simulink model "F16NolinearModel"  (R2013a)
settings: Solver=ode45  StartTime=0.0  StopTime=10  RelTol=1e-3
values from neighbouring files (symbols this model uses):
  alpha0 = trim_state(8)*180/pi    [F16LinmodTestData.m]    (also in F16NolinearModelInitialData.m; F16NolinearModelRemoveWindControlData_low.m = 0; testdata.m)
  b_ref = 9.144    [F16LinmodTestData.m]    (also in F16NolinearModelInitialData.m; F16NolinearModelRemoveWindControlData_low.m = 30; testdata.m = 30)
  dLEF = 0    [F16Data.mat]    (also in F16LinmodTestData.m; F16NolinearModelInitialData.m; F16NolinearModelRemoveWindControlData_low.m; F16hi_7500_394_all.mat)
  fi_flag = 0    [F16LinmodTestData.m]    (also in F16NolinearModelInitialData.m = 1; F16NolinearModelRemoveWindControlData_low.m; testdata.m = 1)
  mass = 636.94*14.59428    (= 9295.6807032)    [F16LinmodTestData.m]    (also in F16NolinearModelInitialData.m; F16NolinearModelRemoveWindControlData_low.m = 636.94; testdata.m = 636.94)
  q = input('Enter the pull-up rate (deg/s):  ')    [trim_F16.m]
  r = input('Enter the turning rate (deg/s):  ')    [trim_F16.m]
  trim_ail = 0.00874607850103852    (= 0.00874607850104)    [F16LinmodTestData.m]    (also in F16NolinearModelInitialData.m; F16NolinearModelRemoveWindControlData_low.m = -1.24450697103e-10; testdata.m; trim_F16.m = UX(4))
  trim_control = [trim_thrust;trim_ele;trim_ail;trim_rud]    [F16LinmodTestData.m]    (also in F16NolinearModelInitialData.m = [trim_thrust,trim_ele,trim_ail,trim_rud]; F16NolinearModelRemoveWindControlData_low.m; runLINF16sim.m = trim_control_lo; testdata.m)
  trim_ele = -2.97973164860638    (= -2.97973164861)    [F16LinmodTestData.m]    (also in F16NolinearModelInitialData.m; F16NolinearModelRemoveWindControlData_low.m = -1.5494258131; testdata.m; trim_F16.m = UX(2))
  trim_rud = 0.0680302158182712    (= 0.0680302158183)    [F16LinmodTestData.m]    (also in F16NolinearModelInitialData.m; F16NolinearModelRemoveWindControlData_low.m = -4.77959844983e-09; testdata.m; trim_F16.m = UX(5))
  trim_thrust = 500    [F16LinmodTestData.m]    (also in F16NolinearModelInitialData.m = 2279.08519955; F16NolinearModelRemoveWindControlData_low.m = -206727.459732; runLINF16sim.m = trim_thrust_lo; testdata.m = 2279.08519955)
  x_cg = 0.09144    [F16LinmodTestData.m]    (also in F16NolinearModelInitialData.m; F16NolinearModelRemoveWindControlData_low.m = 3.962; testdata.m = 3.962)
  x_ref = 0.10668    [F16LinmodTestData.m]    (also in F16NolinearModelInitialData.m; F16NolinearModelRemoveWindControlData_low.m = 3.396; testdata.m = 3.396)
undefined symbols (not defined in the file or in its folder): F, Light, MIL
libraries: aerolibasang x3, aerolibwind2 x3, aerolib6dof2 x1, aerolibconvert2 x1, aerolibatmos2 x1, aerolibgravity2 x1, aerolibadyn x1
settings Model: Creator=Dai  LastModifiedBy=Dai

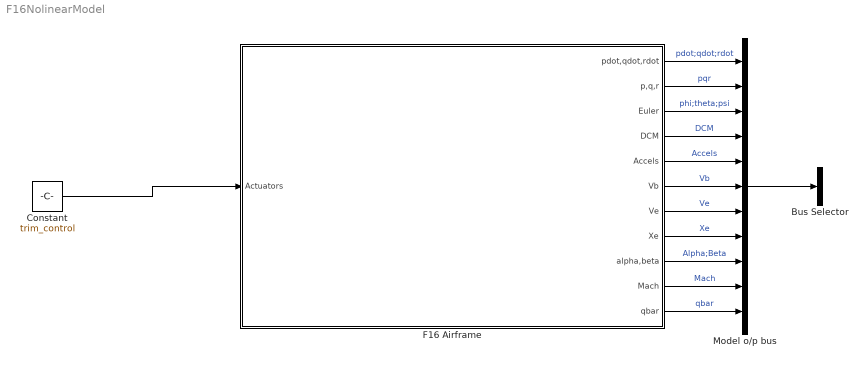
== system F16NolinearModel ==
  Bus Selector : BusSelector  OutputSignals=pdot;qdot;rdot,pqr
  Constant : Constant  Value=trim_control
  F16 Airframe : Subsystem
  Model o/p bus : BusCreator  Inputs=11
  wires:
  F16 Airframe/1(pdot,qdot,rdot) -> Model o/p bus/1  "pdot;qdot;rdot"
  F16 Airframe/2(p,q,r) -> Model o/p bus/2  "pqr"
  F16 Airframe/3(Euler) -> Model o/p bus/3  "phi;theta;psi"
  F16 Airframe/4(DCM) -> Model o/p bus/4  "DCM"
  F16 Airframe/5(Accels) -> Model o/p bus/5  "Accels"
  F16 Airframe/6(Vb) -> Model o/p bus/6  "Vb"
  F16 Airframe/7(Ve) -> Model o/p bus/7  "Ve"
  F16 Airframe/8(Xe) -> Model o/p bus/8  "Xe"
  F16 Airframe/9(alpha,beta) -> Model o/p bus/9  "Alpha;Beta"
  F16 Airframe/10(Mach) -> Model o/p bus/10  "Mach"
  F16 Airframe/11(qbar) -> Model o/p bus/11  "qbar"
  Model o/p bus/1 -> Bus Selector/1
  Constant/1 -> F16 Airframe/1(Actuators)

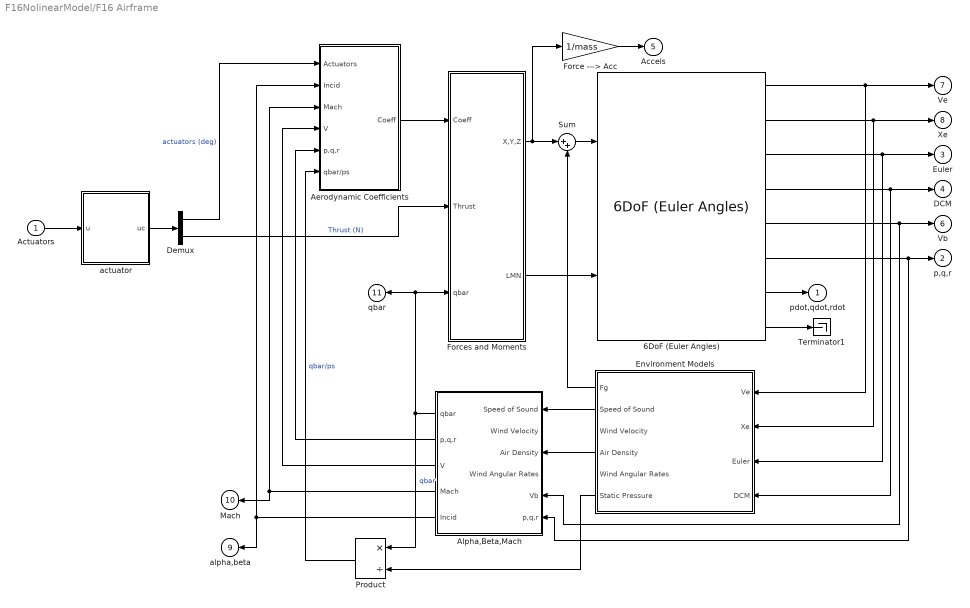
== system F16NolinearModel/F16 Airframe ==
  Actuators : Inport
  6DoF (Euler Angles) : aerolib6dof2/6DoF (Euler Angles)  units=Metric (MKS)  mtype=Fixed  rep=Euler Angles  xme_0=xme_0  Vm_0=Vmw  eul_0=Euler_0  pm_0=pm_0  mass_0=mass  mass_e=0.5  mass_f=2.0  inertia=Inertia  inertia_e=eye(3)  inertia_f=2*eye(3)  k_quat=1.0
  Aerodynamic Coefficients : Subsystem
  Alpha,Beta,Mach : Subsystem
  Demux : Demux  Outputs=2
  Environment Models : Subsystem
  Force ---> Acc : Gain  Gain=1/mass  SaturateOnIntegerOverflow=on  OutDataTypeStr=Inherit: Same as input  ParamDataTypeStr=Inherit: Same as input
  Forces and Moments : Subsystem
  Product : Product  Inputs=*/  SaturateOnIntegerOverflow=on  InputSameDT=on  OutDataTypeStr=Inherit: Same as first input
  Sum : Sum  Inputs=|++  SaturateOnIntegerOverflow=on  InputSameDT=on  OutDataTypeStr=Inherit: Same as first input
  Terminator1 : Terminator
  actuator : Subsystem
  pdot,qdot,rdot : Outport  InitialOutput=0
  p,q,r : Outport  Port=2  InitialOutput=0
  Euler : Outport  Port=3  InitialOutput=0
  DCM : Outport  Port=4  InitialOutput=0
  Accels : Outport  Port=5  InitialOutput=0
  Vb : Outport  Port=6  InitialOutput=0
  Ve : Outport  Port=7  InitialOutput=0
  Xe : Outport  Port=8  InitialOutput=0
  alpha,beta : Outport  Port=9  InitialOutput=0
  Mach : Outport  Port=10  InitialOutput=0
  qbar : Outport  Port=11  InitialOutput=0
  wires:
  6DoF (Euler Angles)/8 -> Terminator1/1
  6DoF (Euler Angles)/1 -> Environment Models/1(Ve), Ve/1
  6DoF (Euler Angles)/2 -> Environment Models/2(Xe), Xe/1
  6DoF (Euler Angles)/6 -> p,q,r/1, Alpha,Beta,Mach/6(p,q,r)
  Demux/2 -> Forces and Moments/2(Thrust)  "Thrust (N)"
  6DoF (Euler Angles)/7 -> pdot,qdot,rdot/1
  6DoF (Euler Angles)/4 -> DCM/1, Environment Models/4(DCM)
  6DoF (Euler Angles)/3 -> Environment Models/3(Euler), Euler/1
  Alpha,Beta,Mach/5(Incid) -> alpha,beta/1, Aerodynamic Coefficients/2(Incid)
  Aerodynamic Coefficients/1(Coeff) -> Forces and Moments/1(Coeff)
  6DoF (Euler Angles)/5 -> Alpha,Beta,Mach/5(Vb), Vb/1
  Environment Models/2(Speed of Sound) -> Alpha,Beta,Mach/1(Speed of Sound)
  Environment Models/4(Air Density) -> Alpha,Beta,Mach/3(Air Density)
  Forces and Moments/2(LMN) -> 6DoF (Euler Angles)/2
  Alpha,Beta,Mach/1(qbar) -> Forces and Moments/3(qbar), qbar/1, Product/1  "qbar"
  Forces and Moments/1(X,Y,Z) -> Force ---> Acc/1, Sum/1
  Sum/1 -> 6DoF (Euler Angles)/1
  Environment Models/1(Fg) -> Sum/2
  Force ---> Acc/1 -> Accels/1
  Alpha,Beta,Mach/3(V) -> Aerodynamic Coefficients/4(V)
  Alpha,Beta,Mach/4(Mach) -> Aerodynamic Coefficients/3(Mach), Mach/1
  Alpha,Beta,Mach/2("p,q,r ") -> Aerodynamic Coefficients/5(p,q,r)
  Environment Models/6(Static Pressure) -> Product/2
  Product/1 -> Aerodynamic Coefficients/6(qbar/ps)  "qbar/ps"
  Actuators/1 -> actuator/1(u)
  actuator/1(uc) -> Demux/1
  Demux/1 -> Aerodynamic Coefficients/1(Actuators)  "actuators (deg)"

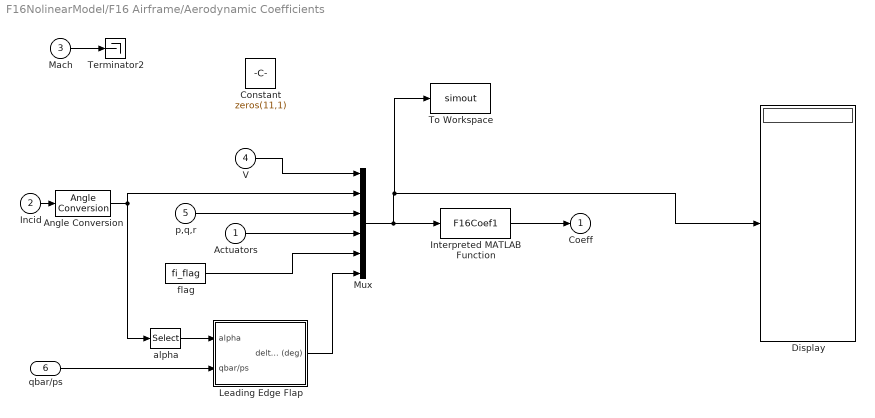
== system F16NolinearModel/F16 Airframe/Aerodynamic Coefficients ==
  Actuators : Inport
  Incid : Inport  Port=2
  Mach : Inport  Port=3
  V : Inport  Port=4
  p,q,r : Inport  Port=5
  qbar/ps : Inport  Port=6
  Angle Conversion : aerolibconvert2/Angle Conversion  IU=rad  OU=deg
  Constant : Constant  Value=zeros(11,1)
  Display : Display
      settings: Decimation=12
  Interpreted MATLAB Function : MATLABFcn  MATLABFcn=F16Coef1  OutputDimensions=6
  Leading Edge Flap : Subsystem
  Mux : Mux  Inputs=6
  Terminator2 : Terminator
  To Workspace : ToWorkspace  VariableName=simout  SampleTime=-1
  alpha : Selector  InputPortWidth=2  IndexOptions=Index vector (dialog)  Indices=1  OutputSizes=1
  flag : Constant  Value=fi_flag
  Coeff : Outport  InitialOutput=0
  wires:
  Angle Conversion/1 -> alpha/1, Mux/2
  Incid/1 -> Angle Conversion/1
  qbar/ps/1 -> Leading Edge Flap/2(qbar/ps)
  alpha/1 -> Leading Edge Flap/1(alpha)
  V/1 -> Mux/1
  p,q,r/1 -> Mux/3
  Actuators/1 -> Mux/4
  flag/1 -> Mux/5
  Mach/1 -> Terminator2/1
  Interpreted MATLAB Function/1 -> Coeff/1
  Mux/1 -> To Workspace/1, Display/1, Interpreted MATLAB Function/1
  Leading Edge Flap/1(delta_lef (deg)) -> Mux/6

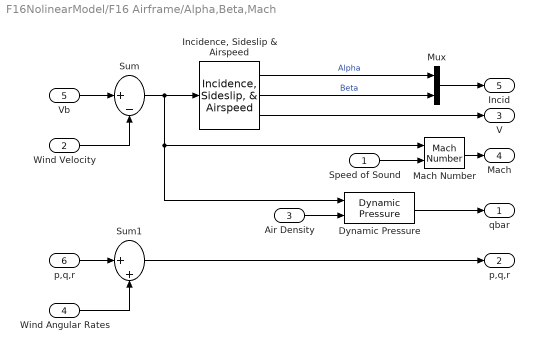
== system F16NolinearModel/F16 Airframe/Alpha,Beta,Mach ==
  Speed of Sound : Inport
  Wind Velocity : Inport  Port=2  PortDimensions=3
  Air Density : Inport  Port=3
  Wind Angular Rates : Inport  Port=4  PortDimensions=3
  Vb : Inport  Port=5  PortDimensions=3
  p,q,r : Inport  Port=6  PortDimensions=3
  Dynamic Pressure : aerolibasang/Dynamic Pressure
  "Incidence, Sideslip & Airspeed" : aerolibasang/Incidence, Sideslip, & Airspeed
  Mach Number : aerolibasang/Mach Number
  Mux : Mux  Inputs=2
  Sum : Sum  Inputs=|+-  SaturateOnIntegerOverflow=on  InputSameDT=on  OutDataTypeStr=Inherit: Same as first input
  Sum1 : Sum  Inputs=|++  SaturateOnIntegerOverflow=on  InputSameDT=on  OutDataTypeStr=Inherit: Same as first input
  qbar : Outport  InitialOutput=0
  "p,q,r " : Outport  Port=2
  V : Outport  Port=3
  Mach : Outport  Port=4
  Incid : Outport  Port=5
  wires:
  "Incidence, Sideslip & Airspeed"/3 -> V/1
  Dynamic Pressure/1 -> qbar/1
  Air Density/1 -> Dynamic Pressure/2
  Mach Number/1 -> Mach/1
  Sum/1 -> Dynamic Pressure/1, Mach Number/1, "Incidence, Sideslip & Airspeed"/1
  Vb/1 -> Sum/1
  Speed of Sound/1 -> Mach Number/2
  Wind Velocity/1 -> Sum/2
  "Incidence, Sideslip & Airspeed"/2 -> Mux/2  "Beta"
  Mux/1 -> Incid/1
  "Incidence, Sideslip & Airspeed"/1 -> Mux/1  "Alpha"
  p,q,r/1 -> Sum1/1
  Wind Angular Rates/1 -> Sum1/2
  Sum1/1 -> "p,q,r "/1

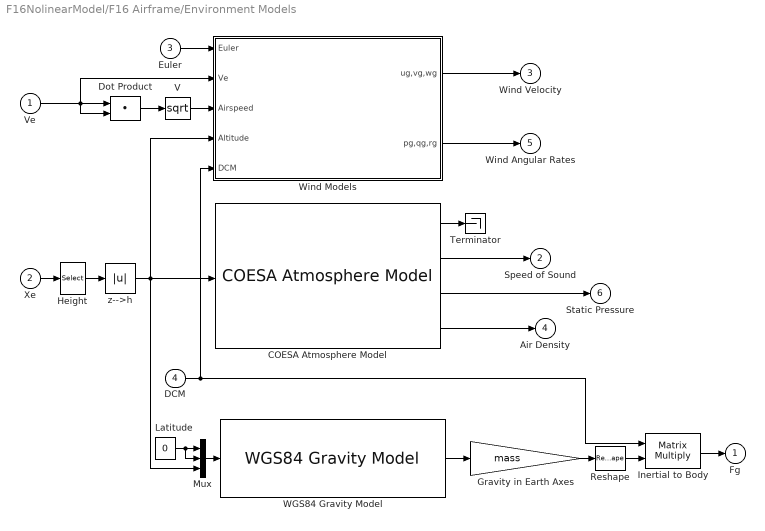
== system F16NolinearModel/F16 Airframe/Environment Models ==
  Ve : Inport
  Xe : Inport  Port=2  PortDimensions=3
  Euler : Inport  Port=3
  DCM : Inport  Port=4
  COESA Atmosphere Model : aerolibatmos2/COESA Atmosphere Model  units=Metric (MKS)  spec=1976 COESA-extended U.S. Standard Atmosphere  model=Profile  profile_var=High temperature  profile_percent=10%  profile_alt=5 km (16404 ft)  envelope_var=High temperature  envelope_percent=1%  action=None
  Dot Product : DotProduct  SaturateOnIntegerOverflow=on  OutDataTypeStr=Inherit: Inherit via internal rule
  Gravity in Earth Axes : Gain  Gain=mass  SaturateOnIntegerOverflow=on  OutDataTypeStr=Inherit: Same as input  ParamDataTypeStr=Inherit: Same as input
  Height : Selector  InputPortWidth=3  IndexOptions=Index vector (dialog)  Indices=[3]  OutputSizes=1
  Inertial to Body : Product  Multiplication=Matrix(*)  SaturateOnIntegerOverflow=on  InputSameDT=on  OutDataTypeStr=Inherit: Same as first input
  Latitude : Constant  Value=0
  Mux : Mux  Inputs=3
  Reshape : Reshape
  Terminator : Terminator
  V : Math  Operator=sqrt  SaturateOnIntegerOverflow=on
  "WGS84 Gravity Model " : aerolibgravity2/WGS84 Gravity Model   model=WGS84 Taylor Series  units=Metric (MKS)  no_atmos=on  precessing=on  jd_loc=off  month=October  day=10  year=2004  no_centrifugal=on  action=None
  Wind Models : Subsystem
  z-->h : Abs  SaturateOnIntegerOverflow=on
  Fg : Outport  InitialOutput=0
  Speed of Sound : Outport  Port=2  InitialOutput=0
  Wind Velocity : Outport  Port=3  InitialOutput=0
  Air Density : Outport  Port=4  InitialOutput=0
  Wind Angular Rates : Outport  Port=5  InitialOutput=0
  Static Pressure : Outport  Port=6
  wires:
  Reshape/1 -> Inertial to Body/2
  Mux/1 -> "WGS84 Gravity Model "/1
  Euler/1 -> Wind Models/1(Euler)
  Ve/1 -> Wind Models/2(Ve), Dot Product/1, Dot Product/2
  Wind Models/1(ug,vg,wg) -> Wind Velocity/1
  Wind Models/2(pg,qg,rg) -> Wind Angular Rates/1
  Dot Product/1 -> V/1
  z-->h/1 -> Mux/3, COESA Atmosphere Model/1, Wind Models/4(Altitude)
  COESA Atmosphere Model/4 -> Air Density/1
  COESA Atmosphere Model/2 -> Speed of Sound/1
  COESA Atmosphere Model/3 -> Static Pressure/1
  COESA Atmosphere Model/1 -> Terminator/1
  Height/1 -> z-->h/1
  Xe/1 -> Height/1
  Latitude/1 -> Mux/2, Mux/1
  "WGS84 Gravity Model "/1 -> Gravity in Earth Axes/1
  Gravity in Earth Axes/1 -> Reshape/1
  DCM/1 -> Wind Models/5(DCM), Inertial to Body/1
  Inertial to Body/1 -> Fg/1
  V/1 -> Wind Models/3(Airspeed)

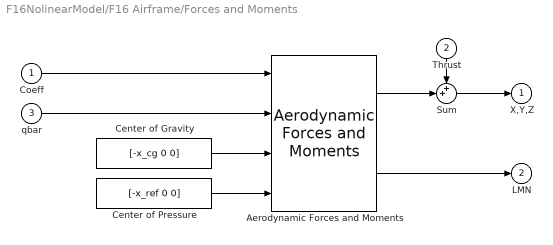
== system F16NolinearModel/F16 Airframe/Forces and Moments ==
  Coeff : Inport
  Thrust : Inport  Port=2
  qbar : Inport  Port=3
  "Aerodynamic Forces and Moments " : aerolibadyn/Aerodynamic Forces and Moments   inputAxes=Body  outputForceAxes=Body  outputMomentAxes=Body  S=S_ref  b=b_ref  cbar=d_ref
  Center of Gravity : Constant  Value=[-x_cg 0 0]
  Center of Pressure : Constant  Value=[-x_ref 0 0]
  Sum : Sum  Inputs=++|  SaturateOnIntegerOverflow=on  InputSameDT=on  OutDataTypeStr=Inherit: Same as first input
  X,Y,Z : Outport  InitialOutput=0
  LMN : Outport  Port=2  InitialOutput=0
  wires:
  Center of Pressure/1 -> "Aerodynamic Forces and Moments "/4
  Center of Gravity/1 -> "Aerodynamic Forces and Moments "/3
  "Aerodynamic Forces and Moments "/1 -> Sum/2
  "Aerodynamic Forces and Moments "/2 -> LMN/1
  Sum/1 -> X,Y,Z/1
  Thrust/1 -> Sum/1
  qbar/1 -> "Aerodynamic Forces and Moments "/2
  Coeff/1 -> "Aerodynamic Forces and Moments "/1

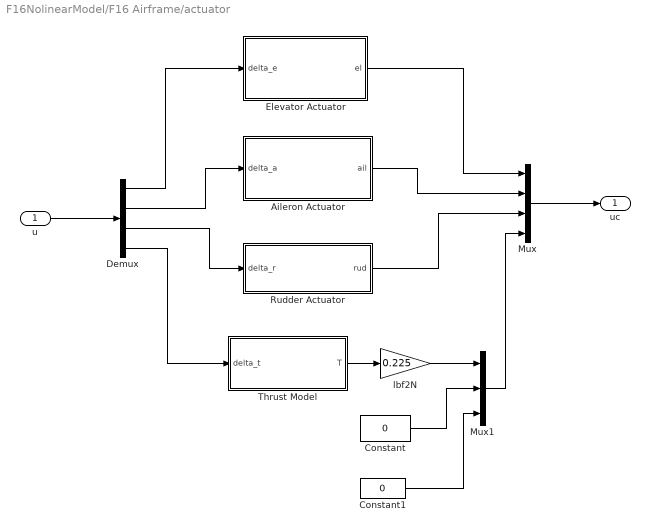
== system F16NolinearModel/F16 Airframe/actuator ==
  u : Inport
  Aileron Actuator : Subsystem
  Constant : Constant  Value=0
  Constant1 : Constant  Value=0
  Demux : Demux
  Elevator Actuator : Subsystem
  Mux : Mux
  Mux1 : Mux  Inputs=3
  Rudder Actuator : Subsystem
  Thrust Model : Subsystem
  lbf2N : Gain  Gain=0.225
  uc : Outport
  wires:
  Demux/3 -> Rudder Actuator/1(delta_r)
  Aileron Actuator/1(ail) -> Mux/2
  Rudder Actuator/1(rud) -> Mux/3
  Demux/2 -> Aileron Actuator/1(delta_a)
  Demux/1 -> Elevator Actuator/1(delta_e)
  Elevator Actuator/1(el) -> Mux/1
  u/1 -> Demux/1
  Demux/4 -> Thrust Model/1(delta_t)
  Thrust Model/1(T) -> lbf2N/1
  Mux/1 -> uc/1
  lbf2N/1 -> Mux1/1
  Constant/1 -> Mux1/2
  Constant1/1 -> Mux1/3
  Mux1/1 -> Mux/4

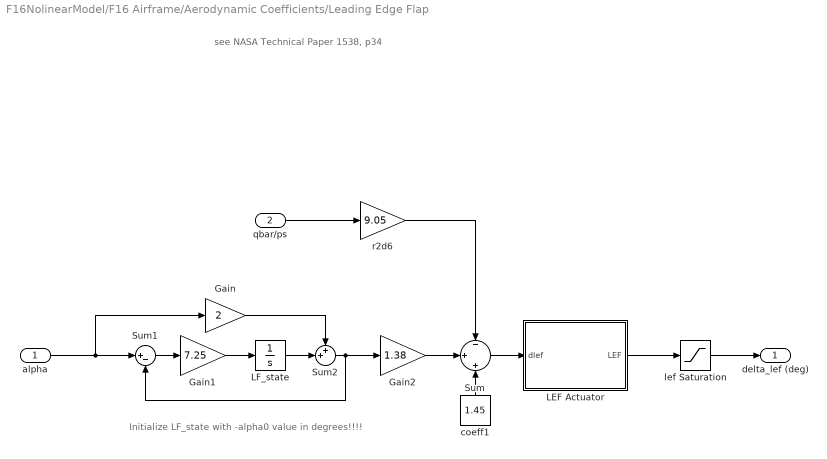
== system F16NolinearModel/F16 Airframe/Aerodynamic Coefficients/Leading Edge Flap ==
  note: see NASA Technical Paper 1538, p34
  note: Initialize LF_state with -alpha0 value in degrees!!!!
  alpha : Inport
  qbar/ps : Inport  Port=2
  Gain : Gain  Gain=2  SaturateOnIntegerOverflow=on  OutDataTypeStr=Inherit: Same as input  ParamDataTypeStr=Inherit: Same as input
  Gain1 : Gain  Gain=7.25  SaturateOnIntegerOverflow=on  OutDataTypeStr=Inherit: Same as input  ParamDataTypeStr=Inherit: Same as input
  Gain2 : Gain  Gain=1.38  SaturateOnIntegerOverflow=on  OutDataTypeStr=Inherit: Same as input  ParamDataTypeStr=Inherit: Same as input
  LEF Actuator : Subsystem
  LF_state : Integrator  InitialCondition=-alpha0
  Sum : Sum  Inputs=-|+|+  SaturateOnIntegerOverflow=on  InputSameDT=on  OutDataTypeStr=Inherit: Same as first input
  Sum1 : Sum  Inputs=|+-  SaturateOnIntegerOverflow=on  InputSameDT=on  OutDataTypeStr=Inherit: Same as first input
  Sum2 : Sum  Inputs=++|  SaturateOnIntegerOverflow=on  InputSameDT=on  OutDataTypeStr=Inherit: Same as first input
  coeff1 : Constant  Value=1.45
  lef Saturation : Saturate  UpperLimit=25  LowerLimit=0
  r2d6 : Gain  Gain=9.05  SaturateOnIntegerOverflow=on  OutDataTypeStr=Inherit: Same as input  ParamDataTypeStr=Inherit: Same as input
  delta_lef (deg) : Outport
  wires:
  Sum1/1 -> Gain1/1
  Gain1/1 -> LF_state/1
  Gain/1 -> Sum2/1
  Gain2/1 -> Sum/2
  coeff1/1 -> Sum/3
  Sum2/1 -> Sum1/2, Gain2/1
  LF_state/1 -> Sum2/2
  alpha/1 -> Sum1/1, Gain/1
  qbar/ps/1 -> r2d6/1
  r2d6/1 -> Sum/1
  lef Saturation/1 -> delta_lef (deg)/1
  Sum/1 -> LEF Actuator/1(dlef)
  LEF Actuator/1(LEF) -> lef Saturation/1

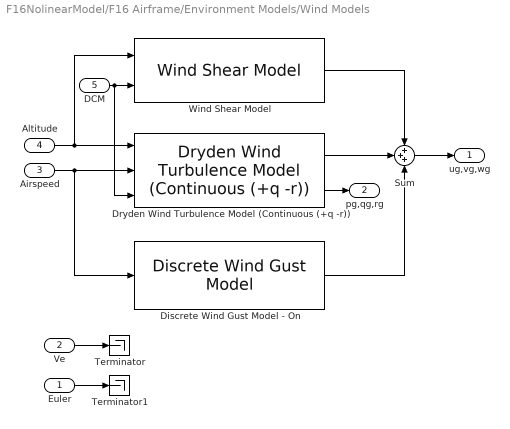
== system F16NolinearModel/F16 Airframe/Environment Models/Wind Models ==
  Euler : Inport
  Ve : Inport  Port=2
  Airspeed : Inport  Port=3
  Altitude : Inport  Port=4
  DCM : Inport  Port=5
  Discrete Wind Gust Model - On : aerolibwind2/Discrete Wind Gust Model  units=Metric (MKS)  Gx=on  Gy=on  Gz=on  t_0=20  d_m=[120 120 80]  v_m=[3.5 3.0 3.0]
  Dryden Wind Turbulence Model (Continuous (+q -r)) : aerolibwind2/Dryden Wind Turbulence Model  (Continuous (+q -r))  units=Metric (MKS)  spec=MIL-F-8785C  model=Continuous Dryden (+q -r)  W20=5  Wdeg=0  TurbProb=10^-2 - Light  L_high=533.4  Wingspan=4  ts=0.1  Seed=[23341 23342 23343 23344]  T_on=on
  Sum : Sum  Inputs=+++  SaturateOnIntegerOverflow=on  InputSameDT=on  OutDataTypeStr=Inherit: Same as first input
  Terminator : Terminator
  Terminator1 : Terminator
  Wind Shear Model : aerolibwind2/Wind Shear Model  units=Metric (MKS)  phase=Category C - Terminal Flight Phase  W_20=1  Wdeg=0
  ug,vg,wg : Outport
  pg,qg,rg : Outport  Port=2
  wires:
  Euler/1 -> Terminator1/1
  Ve/1 -> Terminator/1
  Wind Shear Model/1 -> Sum/1
  Dryden Wind Turbulence Model (Continuous (+q -r))/1 -> Sum/2
  Discrete Wind Gust Model - On/1 -> Sum/3
  Sum/1 -> ug,vg,wg/1
  DCM/1 -> Dryden Wind Turbulence Model (Continuous (+q -r))/3, Wind Shear Model/2
  Airspeed/1 -> Dryden Wind Turbulence Model (Continuous (+q -r))/2, Discrete Wind Gust Model - On/1
  Dryden Wind Turbulence Model (Continuous (+q -r))/2 -> pg,qg,rg/1
  Altitude/1 -> Dryden Wind Turbulence Model (Continuous (+q -r))/1, Wind Shear Model/1

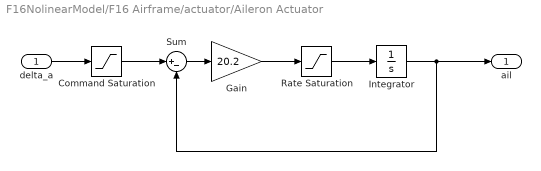
== system F16NolinearModel/F16 Airframe/actuator/Aileron Actuator ==
  delta_a : Inport
  Command Saturation : Saturate  UpperLimit=21.5  LowerLimit=-21.5
  Gain : Gain  Gain=20.2  SaturateOnIntegerOverflow=on  OutDataTypeStr=Inherit: Same as input  ParamDataTypeStr=Inherit: Same as input
  "Integrator " : Integrator  InitialCondition=trim_ail  UpperSaturationLimit=21.5  LowerSaturationLimit=-21.5
  Rate Saturation : Saturate  UpperLimit=80  LowerLimit=-80
  Sum : Sum  Inputs=|+-  SaturateOnIntegerOverflow=on  InputSameDT=on  OutDataTypeStr=Inherit: Same as first input
  ail : Outport
  wires:
  delta_a/1 -> Command Saturation/1
  "Integrator "/1 -> ail/1, Sum/2
  Sum/1 -> Gain/1
  Gain/1 -> Rate Saturation/1
  Command Saturation/1 -> Sum/1
  Rate Saturation/1 -> "Integrator "/1

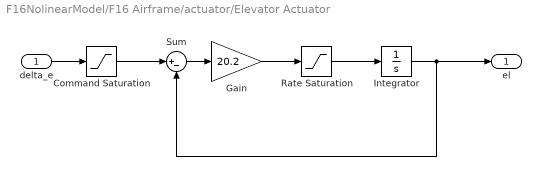
== system F16NolinearModel/F16 Airframe/actuator/Elevator Actuator ==
  delta_e : Inport
  Command Saturation : Saturate  UpperLimit=25  LowerLimit=-25
  Gain : Gain  Gain=20.2  SaturateOnIntegerOverflow=on  OutDataTypeStr=Inherit: Same as input  ParamDataTypeStr=Inherit: Same as input
  "Integrator " : Integrator  InitialCondition=trim_ele  UpperSaturationLimit=25  LowerSaturationLimit=-25
  Rate Saturation : Saturate  UpperLimit=60  LowerLimit=-60
  Sum : Sum  Inputs=|+-  SaturateOnIntegerOverflow=on  InputSameDT=on  OutDataTypeStr=Inherit: Same as first input
  el : Outport
  wires:
  delta_e/1 -> Command Saturation/1
  Command Saturation/1 -> Sum/1
  Sum/1 -> Gain/1
  Gain/1 -> Rate Saturation/1
  "Integrator "/1 -> el/1, Sum/2
  Rate Saturation/1 -> "Integrator "/1

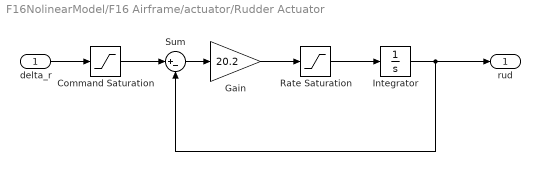
== system F16NolinearModel/F16 Airframe/actuator/Rudder Actuator ==
  delta_r : Inport
  Command Saturation : Saturate  UpperLimit=30  LowerLimit=-30
  Gain : Gain  Gain=20.2  SaturateOnIntegerOverflow=on  OutDataTypeStr=Inherit: Same as input  ParamDataTypeStr=Inherit: Same as input
  "Integrator " : Integrator  InitialCondition=trim_rud  UpperSaturationLimit=30  LowerSaturationLimit=-30
  Rate Saturation : Saturate  UpperLimit=120  LowerLimit=-120
  Sum : Sum  Inputs=|+-  SaturateOnIntegerOverflow=on  InputSameDT=on  OutDataTypeStr=Inherit: Same as first input
  rud : Outport
  wires:
  "Integrator "/1 -> rud/1, Sum/2
  Sum/1 -> Gain/1
  delta_r/1 -> Command Saturation/1
  Rate Saturation/1 -> "Integrator "/1
  Gain/1 -> Rate Saturation/1
  Command Saturation/1 -> Sum/1

== system F16NolinearModel/F16 Airframe/actuator/Thrust Model ==
  delta_t : Inport
  Command Saturation : Saturate  UpperLimit=19000  LowerLimit=1000
  Gain : Gain  SaturateOnIntegerOverflow=on  OutDataTypeStr=Inherit: Same as input  ParamDataTypeStr=Inherit: Same as input
  "Integrator " : Integrator  InitialCondition=trim_thrust  UpperSaturationLimit=30  LowerSaturationLimit=-30
  Rate Saturation : Saturate  UpperLimit=10000  LowerLimit=-10000
  Sum : Sum  Inputs=|+-  SaturateOnIntegerOverflow=on  InputSameDT=on  OutDataTypeStr=Inherit: Same as first input
  T : Outport
  wires:
  delta_t/1 -> Command Saturation/1
  Gain/1 -> Rate Saturation/1
  "Integrator "/1 -> T/1, Sum/2
  Command Saturation/1 -> Sum/1
  Sum/1 -> Gain/1
  Rate Saturation/1 -> "Integrator "/1

== system F16NolinearModel/F16 Airframe/Aerodynamic Coefficients/Leading Edge Flap/LEF Actuator ==
  dlef : Inport
  Command Saturation : Saturate  UpperLimit=25  LowerLimit=0
  Gain3 : Gain  Gain=1/0.136  SaturateOnIntegerOverflow=on  OutDataTypeStr=Inherit: Same as input  ParamDataTypeStr=Inherit: Same as input
  "Integrator " : Integrator  InitialCondition=dLEF  UpperSaturationLimit=21.5  LowerSaturationLimit=-21.5
  Rate Saturation : Saturate  UpperLimit=25  LowerLimit=-25
  Sum3 : Sum  Inputs=|+-  SaturateOnIntegerOverflow=on  InputSameDT=on  OutDataTypeStr=Inherit: Same as first input
  LEF : Outport
  wires:
  Gain3/1 -> Rate Saturation/1
  Rate Saturation/1 -> "Integrator "/1
  "Integrator "/1 -> LEF/1, Sum3/2
  Sum3/1 -> Gain3/1
  dlef/1 -> Command Saturation/1
  Command Saturation/1 -> Sum3/1
